simulink subsystem "traction"  (R2024b)
settings: Solver=VariableStepAuto  StartTime=0.0  StopTime=10.0  RelTol=1e-3
settings Model: Creator=yevge  LastModifiedBy=yevge

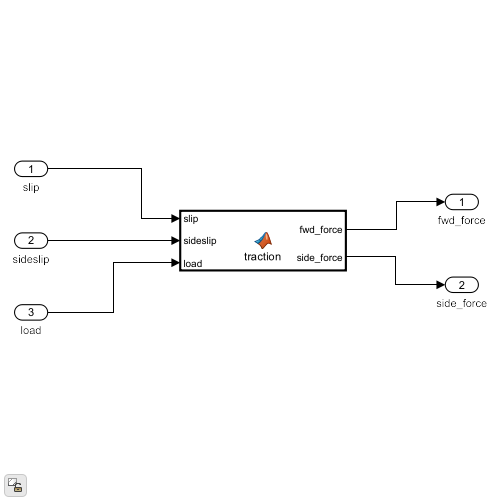
[thumbnail: Simulink's stored preview of the top-level diagram]
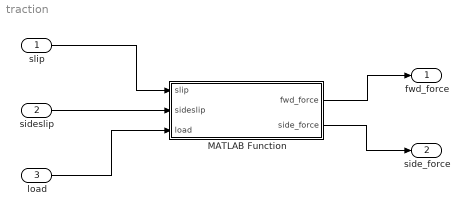
== system traction ==
  slip : Inport  Unit=1  PortDimensions=1
  sideslip : Inport  Port=2  Unit=rad  PortDimensions=1
  load : Inport  Port=3  Unit=N  PortDimensions=1
  MATLAB Function : MATLAB Function  TreatAsAtomicUnit=on
  fwd_force : Outport  Unit=N  PortDimensions=1
  side_force : Outport  Port=2  Unit=N  PortDimensions=1
  wires:
  load/1 -> MATLAB Function/3(load)
  slip/1 -> MATLAB Function/1(slip)
  sideslip/1 -> MATLAB Function/2(sideslip)
  MATLAB Function/1(fwd_force) -> fwd_force/1
  MATLAB Function/2(side_force) -> side_force/1

== matlab function traction/MATLAB Function ==
  data: slip input; fwd_force output; sideslip input; load input; side_force output
function [fwd_force, side_force] = traction(slip, sideslip, load) 
    fwd_force = sin(atan(slip)) * load;
    side_force = sin(sideslip) * load;
end
